simulink model "SolarcellEnergy"  (R2015b)
settings: Solver=VariableStepAuto  StartTime=0.0  StopTime=43200  RelTol=1e-3
model workspace (MAT data in the model file):
  ans = 14
  area = 20
  eta = 0.22
  max_irradiance = Simulink.Parameter
  max_irradiance.Value = 542
  max_irradiance.DataType = 'auto'
  max_irradiance.Units = 'auto'
settings Model: Creator=aemili  LastModifiedBy=aemili

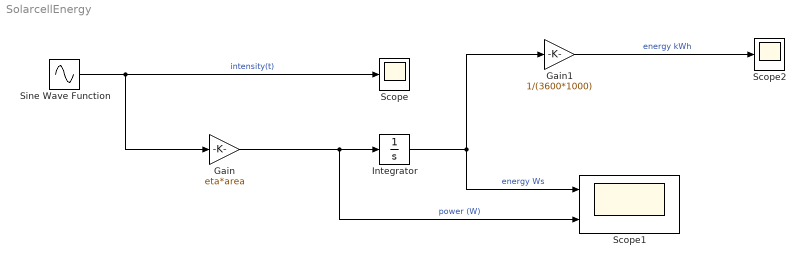
== system SolarcellEnergy ==
  Gain : Gain  Gain=eta*area
  Gain1 : Gain  Gain=1/(3600*1000)
  Integrator : Integrator
  Scope : Scope
  Scope1 : Scope  NumInputPorts=2
  Scope2 : Scope
  Sine Wave Function : Sin  Amplitude=max_irradiance  Frequency=(pi/(12*3600))  SampleTime=0
  wires:
  Sine Wave Function/1 -> Gain/1, Scope/1  "intensity(t)"
  Gain/1 -> Scope1/2, Integrator/1  "power (W)"
  Integrator/1 -> Gain1/1, Scope1/1  "energy Ws"
  Gain1/1 -> Scope2/1  "energy kWh"
